simulink model "sim_main_esb_12_modGAMC_Int2_LG"  (Simulink 8.9)
settings: Solver=VariableStepAuto  StartTime=0.0  StopTime=10  RelTol=1e-3
values from neighbouring files (symbols this model uses):
  A = 0.914    [KALMAN.m]    (also in main_cntl.m = eval(A_eq); main_sys.m = double(A_lin); main_sys_klm.m = double(A_lin); main_tf_0.m = A)
  B = 0.25    [KALMAN.m]    (also in main_cntl.m = eval(B_eq); main_sys.m = double(B_lin); main_sys_klm.m = double(B_lin); main_tf_1.m = eval(B))
  C = 0.344    [KALMAN.m]    (also in main_sys.m = double( subs( C) ); main_sys_klm.m = double( subs( C) ); main_tf_0.m = [ 0 , 0  , Ks , ds , -Ks , -ds, 0 ]; main_tf_1.m = C_mes)
  Ct = double( subs( Ct) )    [main_sys.m]    (also in main_sys_klm.m; main_tf_10.m; main_tf_11.m; main_tf_12.m)
  D = zeros(7,2)    [main_sys.m]    (also in main_sys_klm.m = zeros(2,2); main_tf_0.m = [ 0 , 0 ]; main_tf_1.m = zeros(1,1); main_tf_10.m = zeros(2,2))
  sys_sys = ss(A,B,C,D)    [main_sys.m]    (also in main_sys_klm.m; main_tf_10.m; main_tf_11.m; main_tf_12.m = ss(A_sys,B_sys,C_sys_mod,D_sys_mod))
undefined symbols (not defined in the file or in its folder): Continuous, K_lq3, Time
libraries: ctrlSharedLib x1
settings Model: Creator=eshojaei  LastModifiedBy=Gustavo
settings DataIOCC: LimitDataPoints=off  SaveFormat=Dataset  SignalLoggingSaveFormat=Dataset
settings OptimizationCC: LifeSpan=auto
settings DebuggingCC: UnderspecifiedInitializationDetection=Simplified  MergeDetectMultiDrivingBlocksExec=error  FcnCallInpInsideContextMsg=error  StateNameClashWarn=none  SFUnexpectedBacktrackingDiag=error  SFNoUnconditionalDefaultTransitionDiag=error  SFExecutionAtInitializationDiag=warning
settings HardwareCC: ProdBitPerPointer=64  ProdBitPerSizeT=64  ProdBitPerPtrDiffT=64  ProdLargestAtomicFloat=Float  ProdIntDivRoundTo=Zero  ProdEndianess=LittleEndian  ProdWordSize=64  ProdHWDeviceType=Intel->x86-64 (Windows64)
settings ModelReferenceCC: PropagateSignalLabelsOutOfModel=on
settings SFSimCC: SimUseLocalCustomCode=on
settings RTWCC: RTWUseLocalCustomCode=on
settings GRTTargetCC: TargetLangStandard=C99 (ISO)  GeneratePreprocessorConditionals=Use local settings  CombineOutputUpdateFcns=on  GRTInterface=off
settings ConfigComp: CovMetricSettings=dwe  CovHtmlReporting=off  CovSaveCumulativeToWorkspaceVar=off  CovSaveSingleToWorkspaceVar=off  CovExternalEMLEnable=on

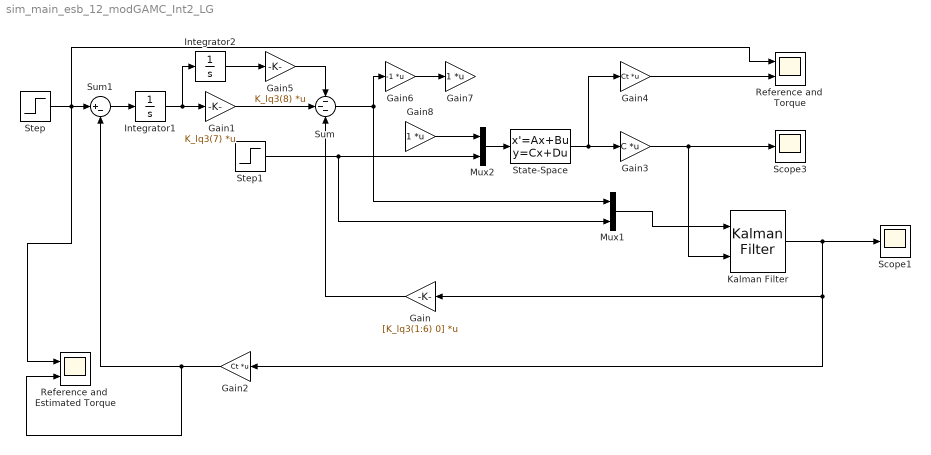
== system sim_main_esb_12_modGAMC_Int2_LG ==
  Gain : Gain  Gain=[K_lq3(1:6) 0]  Multiplication=Matrix(K*u)
  Gain1 : Gain  Gain=K_lq3(7)  Multiplication=Matrix(K*u)
  Gain2 : Gain  Gain=Ct  Multiplication=Matrix(K*u)
  Gain3 : Gain  Gain=C  Multiplication=Matrix(K*u)
  Gain4 : Gain  Gain=Ct  Multiplication=Matrix(K*u)
  Gain5 : Gain  Gain=K_lq3(8)  Multiplication=Matrix(K*u)
  Gain6 : Gain  Gain=-1  Multiplication=Matrix(K*u)
  Gain7 : Gain  Multiplication=Matrix(K*u)
  Gain8 : Gain  Multiplication=Matrix(K*u)
  Integrator1 : Integrator
  Integrator2 : Integrator
  Kalman Filter : ctrlSharedLib/Kalman Filter  TimeDomain=Continuous-Time  UseCurrentEstimator=on  ModelSource=Individual A, B, C, D matrices  ModelSourceVariable=ss(0.95,1,1,0,1)  A=A  B=B  C=C  D=D  NumberOfStates=1  NumberOfInputs=1  NumberOfOutputs=1  InitialEstimateSource=Dialog  X0=0  P0=10  UseK=off  UseGH=off  NumberOfProcessNoiseInputs=1  G=1  TimeInvariantG=on  H=0  TimeInvariantH=on  Q=0.05  TimeInvariantQ=on  R=1  TimeInvariantR=on  N=0  TimeInvariantN=on  AddInputPort=on  AddEnablePort=off  ExternalReset=none  OutputEstimatedY=off  OutputP=off  Ts=-1
      settings: SourceProductBaseCode=CT
  Mux1 : Mux  Inputs=2
  Mux2 : Mux  Inputs=2
  Reference and  Estimated Torque : Scope  NumInputPorts=2
  Reference and  Torque : Scope  NumInputPorts=2
  Scope1 : Scope
  Scope3 : Scope
  State-Space : StateSpace  A=sys_sys.A  B=sys_sys.B  C=sys_sys.C  D=sys_sys.D  X0=0
  Step : Step  Time=.1  After=10  SampleTime=0
  Step1 : Step  Time=.1  After=.1  SampleTime=0
  Sum : Sum  Inputs=---
  Sum1 : Sum  Inputs=|+-
  wires:
  Integrator1/1 -> Integrator2/1, Gain1/1
  Sum1/1 -> Integrator1/1
  Step1/1 -> Mux2/2, Mux1/2
  Gain3/1 -> Scope3/1, Kalman Filter/2
  State-Space/1 -> Gain3/1, Gain4/1
  Gain4/1 -> Reference and  Torque/2
  Mux1/1 -> Kalman Filter/1
  Mux2/1 -> State-Space/1
  Sum/1 -> Gain6/1, Mux1/1
  Kalman Filter/1 -> Gain2/1, Gain/1, Scope1/1
  Integrator2/1 -> Gain5/1
  Gain/1 -> Sum/3
  Gain1/1 -> Sum/2
  Gain5/1 -> Sum/1
  Gain2/1 -> Reference and  Estimated Torque/2, Sum1/2
  Step/1 -> Reference and  Estimated Torque/1, Reference and  Torque/1, Sum1/1
  Gain6/1 -> Gain7/1
  Gain8/1 -> Mux2/1
